simulink model "Proyecto_final_itae"  (R2020a)
settings: Solver=VariableStepAuto  StartTime=0.0  StopTime=10.0  RelTol=1e-3
values from neighbouring files (symbols this model uses):
  A = [0 0 1 0 ... (first row only)    [itaeosts.m]
  B = [0;0;(Kg*Ki*n_total)/(Rm*(Jb+mb*delta_2^2)*((L/d)));0]    [itaeosts.m]
  C = [0 1 0 0]    [itaeosts.m]
  D = 0    [itaeosts.m]
  L = 0.425    [itaeosts.m]
undefined symbols (not defined in the file or in its folder): K_itae, Kext_itae, Kp_itae, rank, sysobs_cl_itae, sysobs_itae, sysobsext_itae
settings Model: Creator=Windows_10  LastModifiedBy=Windows_10

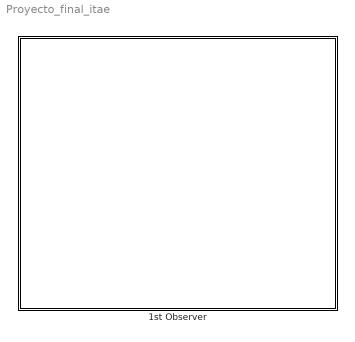
== system Proyecto_final_itae ==
  1st Observer : Subsystem

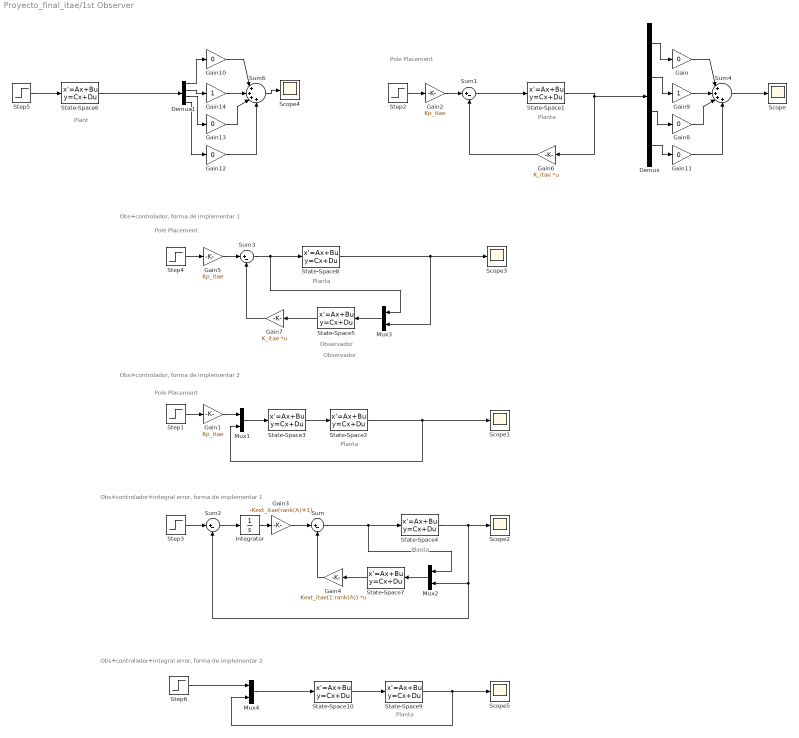
== system Proyecto_final_itae/1st Observer ==
  note: Planta
  note: Planta
  note: Planta
  note: Planta
  note: Planta
  note: Plant
  note: Obs+controlador+integral error, forma de implementar 1
  note: Observador
  note: Pole Placement
  note: Pole Placement
  note: Observador
  note: Pole Placement
  note: Obs+controlador, forma de implementar 1
  note: Obs+controlador, forma de implementar 2
  note: Obs+controlador+integral error, forma de implementar 2
  Demux : Demux
  Demux1 : Demux
  Gain{,8,10..13} (6 alike) : Gain  Gain=0
  Gain1 : Gain  Gain=Kp_itae
  Gain14 : Gain
  Gain2 : Gain  Gain=Kp_itae
  Gain3 : Gain  Gain=-Kext_itae(rank(A)+1)
  Gain4 : Gain  Gain=Kext_itae(1:rank(A))  Multiplication=Matrix(K*u)
  Gain5 : Gain  Gain=Kp_itae
  Gain6 : Gain  Gain=K_itae  Multiplication=Matrix(K*u)
  Gain7 : Gain  Gain=K_itae  Multiplication=Matrix(K*u)
  Gain9 : Gain
  Integrator : Integrator
  Mux{1..4} (4 alike) : Mux  Inputs=2
  Scope{,1..5} (6 alike) : Scope
  State-Space1 : StateSpace  A=A  B=B  C=eye(rank(A))  D=zeros(rank(A),1)  InitialCondition=0
  State-Space10 : StateSpace  A=sysobsext_itae.A  B=sysobsext_itae.B  C=sysobsext_itae.C  D=sysobsext_itae.D  InitialCondition=0
  State-Space{2,4,8..9} (4 alike) : StateSpace  A=A  B=B  C=C  D=D  InitialCondition=0
  State-Space3 : StateSpace  A=sysobs_cl_itae.A  B=sysobs_cl_itae.B  C=sysobs_cl_itae.C  D=sysobs_cl_itae.D  InitialCondition=0
  State-Space5 : StateSpace  A=sysobs_itae.A  B=sysobs_itae.B  C=sysobs_itae.C  D=sysobs_itae.D  InitialCondition=0
  State-Space6 : StateSpace  A=A  B=B  C=eye(rank(A))  D=zeros(rank(A),1)  InitialCondition=0
  State-Space7 : StateSpace  A=sysobs_itae.A  B=sysobs_itae.B  C=sysobs_itae.C  D=sysobs_itae.D  InitialCondition=0
  Step{1..3,5..6} (5 alike) : Step  Time=0  SampleTime=0
  Step4 : Step  Time=0  After=L/2  SampleTime=0
  Sum{,1..3} (4 alike) : Sum  Inputs=|+-
  Sum4 : Sum  Inputs=|++++
  Sum6 : Sum  Inputs=|++++
  wires:
  Gain4/1 -> Sum/2
  Gain7/1 -> Sum3/2
  Gain6/1 -> Sum1/2
  State-Space2/1 -> Mux1/2, Scope1/1
  Sum/1 -> State-Space4/1, Mux2/1
  Demux1/2 -> Gain14/1
  State-Space3/1 -> State-Space2/1
  Demux1/3 -> Gain13/1
  Demux/2 -> Gain9/1
  Gain1/1 -> Mux1/1
  Gain13/1 -> Sum6/3
  Step3/1 -> Sum2/1
  Mux1/1 -> State-Space3/1
  State-Space5/1 -> Gain7/1
  Step4/1 -> Gain5/1
  Step5/1 -> State-Space6/1
  Gain5/1 -> Sum3/1
  Sum1/1 -> State-Space1/1
  State-Space4/1 -> Sum2/2, Mux2/2, Scope2/1
  Mux3/1 -> State-Space5/1
  Sum3/1 -> Mux3/1, State-Space8/1
  Gain2/1 -> Sum1/1
  State-Space8/1 -> Scope3/1, Mux3/2
  Mux4/1 -> State-Space10/1
  Demux/1 -> Gain/1
  Mux2/1 -> State-Space7/1
  State-Space7/1 -> Gain4/1
  Step2/1 -> Gain2/1
  Gain/1 -> Sum4/1
  Step6/1 -> Mux4/1
  Demux1/1 -> Gain10/1
  Sum2/1 -> Integrator/1
  State-Space6/1 -> Demux1/1
  Step1/1 -> Gain1/1
  Gain10/1 -> Sum6/1
  Gain3/1 -> Sum/1
  Integrator/1 -> Gain3/1
  State-Space1/1 -> Demux/1, Gain6/1
  State-Space9/1 -> Mux4/2, Scope5/1
  Gain8/1 -> Sum4/3
  Sum6/1 -> Scope4/1
  Gain14/1 -> Sum6/2
  Gain9/1 -> Sum4/2
  Sum4/1 -> Scope/1
  Demux/3 -> Gain8/1
  State-Space10/1 -> State-Space9/1
  Demux/4 -> Gain11/1
  Gain11/1 -> Sum4/4
  Demux1/4 -> Gain12/1
  Gain12/1 -> Sum6/4
